simulink model "two_tone_test_2020b"  (R2020b)
settings: Solver=VariableStepDiscrete  StartTime=0.0  StopTime=1000.5  RelTol=1e-3  EnableMultiTasking=on
PreLoadFcn:
  | A=sqrt(1e-3);
  | a1=10;
  | IIP3=15;
libraries: commrflib2 x1
settings Model: Creator=professor  LastModifiedBy=14083
settings DataIOCC: LimitDataPoints=on  SaveFormat=Array  SignalLoggingSaveFormat=ModelDataLogs  ReturnWorkspaceOutputs=off
settings OptimizationCC: ExpressionDepthLimit=2147483647  InitFltsAndDblsToZero=on  LifeSpan=inf
settings DebuggingCC: UnderspecifiedInitializationDetection=Classic  MergeDetectMultiDrivingBlocksExec=none  SolverPrmCheckMsg=warning  MultiTaskDSMMsg=warning  MultiTaskCondExecSysMsg=none  FcnCallInpInsideContextMsg=warning  StateNameClashWarn=warning  SFUnexpectedBacktrackingDiag=warning  SFNoUnconditionalDefaultTransitionDiag=warning  SFExecutionAtInitializationDiag=none  ArithmeticOperatorsInVariantConditions=warning
settings HardwareCC: ProdBitPerPointer=32  ProdBitPerSizeT=32  ProdBitPerPtrDiffT=32  ProdLargestAtomicFloat=None  ProdIntDivRoundTo=Undefined  ProdEndianess=Unspecified  ProdWordSize=32  ProdHWDeviceType=32-bit Generic  TargetHWDeviceType=32-bit Generic
settings ModelReferenceCC: PropagateSignalLabelsOutOfModel=off
settings SFSimCC: SimUseLocalCustomCode=off  CustomCodeUndefinedFunction=UseInterfaceOnly
settings RTWCC: RTWUseLocalCustomCode=off
settings CodeAppCC: StateflowObjectComments=on
settings GRTTargetCC: TargetFcnLib=ansi_tfl_tmw.mat  TargetLangStandard=C89/C90 (ANSI)  CombineOutputUpdateFcns=off  GRTInterface=on
settings ConfigComp: CovMetricSettings=dw  CovSaveCumulativeToWorkspaceVar=on  CovSaveSingleToWorkspaceVar=on  CovExternalEMLEnable=off

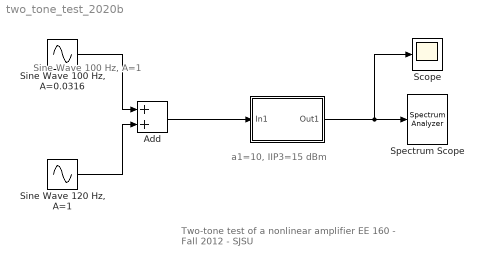
== system two_tone_test_2020b ==
  note: Two-tone test of a nonlinear amplifier
      | EE 160 - Fall 2012 - SJSU
  note: a1=10, IIP3=15 dBm
  note: Sine Wave
      | 100 Hz, A=1
  " " : Subsystem
      mask Display: disp('Nonlinear\nAmplifier')
  Add : Sum
  Scope : Scope
  "Sine Wave 100 Hz, A=0.0316" : Sin  Amplitude=A  Frequency=2*pi*100  SampleTime=1/440
  "Sine Wave 120 Hz, A=1" : Sin  Amplitude=A  Frequency=2*pi*120  SampleTime=1/440
  Spectrum Scope : SpectrumAnalyzer
  wires:
  Add/1 -> " "/1(In1)
  "Sine Wave 100 Hz, A=0.0316"/1 -> Add/1
  "Sine Wave 120 Hz, A=1"/1 -> Add/2
  " "/1(Out1) -> Scope/1, Spectrum Scope/1

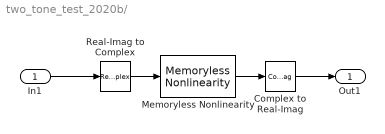
== system two_tone_test_2020b/  ==
  In1 : Inport
  Complex to Real-Imag : ComplexToRealImag  Output=Real
  Memoryless Nonlinearity : commrflib2/Memoryless Nonlinearity  model_select=Hyperbolic tangent  linGaindB=a1  GindB=0  iip3=IIP3  am2pm=0  LPwrLimAMPM=0  UPwrLimAMPM=50  amam=[2.1587 1.1517]  ampm=[4.0033 9.1040]  x=[8.1081 1.5413 6.5202 -0.0718]  y=[4.6645 2.0965 10.88 -0.003]  p=0.5  GoutdB=0  vsat=1
      settings: SourceProductBaseCode=CM
  Real-Imag to Complex : RealImagToComplex  Input=Real
  Out1 : Outport  VectorParamsAs1DForOutWhenUnconnected=off
  wires:
  Memoryless Nonlinearity/1 -> Complex to Real-Imag/1
  Real-Imag to Complex/1 -> Memoryless Nonlinearity/1
  Complex to Real-Imag/1 -> Out1/1
  In1/1 -> Real-Imag to Complex/1
